simulink model "SSB_FilterMethod"  (R2021a)
settings: Solver=VariableStepAuto  StartTime=0.0  StopTime=10.0  RelTol=1e-3
libraries: dspfdesign x2
settings Model: Creator=ZephyrY  LastModifiedBy=ZephyrY

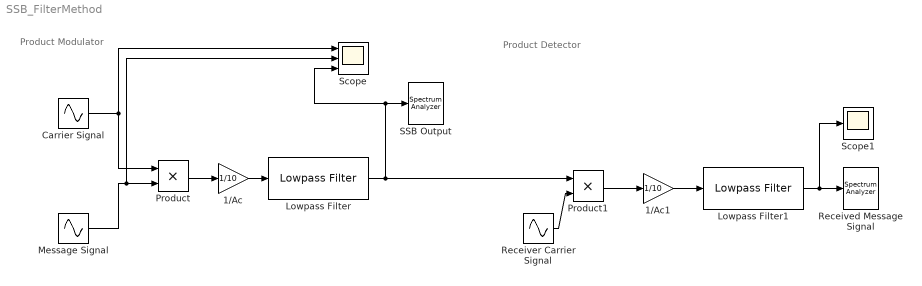
== system SSB_FilterMethod ==
  note: Product Detector
  note: Product Modulator
  1/Ac : Gain  Gain=1/10
  1/Ac1 : Gain  Gain=1/10
  Carrier Signal : Sin  Amplitude=10  Frequency=2*pi*100  Phase=pi/2  SampleTime=1e-3
  Lowpass Filter : dspfdesign/Lowpass Filter  FilterType=FIR  DesignForMinimumOrder=off  FilterOrder=200  PassbandFrequency=93  StopbandFrequency=12e3  PassbandRipple=0.1  StopbandAttenuation=80  InheritSampleRate=on  SampleRate=44100  SimulateUsing=Interpreted execution  roundingMode=Floor  coeffsDataTypeStr=fixdt(1,16)
  Lowpass Filter1 : dspfdesign/Lowpass Filter  FilterType=FIR  DesignForMinimumOrder=off  FilterOrder=200  PassbandFrequency=13  StopbandFrequency=12e3  PassbandRipple=0.1  StopbandAttenuation=80  InheritSampleRate=on  SampleRate=44100  SimulateUsing=Interpreted execution  roundingMode=Floor  coeffsDataTypeStr=fixdt(1,16)
  Message Signal : Sin  Amplitude=5  Frequency=2*pi*10  Phase=pi/2  SampleTime=1e-3
  Product : Product
  Product1 : Product
  Received Message Signal : SpectrumAnalyzer
  Receiver Carrier Signal : Sin  Amplitude=10  Frequency=2*pi*100  Phase=pi/2  SampleTime=1e-3
  SSB Output : SpectrumAnalyzer
  Scope : Scope  NumInputPorts=3
  Scope1 : Scope
  wires:
  Message Signal/1 -> Scope/2, Product/2
  1/Ac/1 -> Lowpass Filter/1
  Carrier Signal/1 -> Scope/1, Product/1
  Product/1 -> 1/Ac/1
  Lowpass Filter/1 -> Product1/1, Scope/3, SSB Output/1
  Receiver Carrier Signal/1 -> Product1/2
  Product1/1 -> 1/Ac1/1
  Lowpass Filter1/1 -> Scope1/1, Received Message Signal/1
  1/Ac1/1 -> Lowpass Filter1/1
